simulink model "model_groundTethered"  (R2015b)
settings: Solver=ode45  StartTime=0.0  StopTime=T_sim  FixedStep=dt  RelTol=1e-3
PreLoadFcn:
  | setup;
InitFcn:
  | setup;
StartFcn:
  | setup;
values from neighbouring files (symbols this model uses):
  A_act = [-100 0 0 0 0 -100 0 0 0 0 -100 0 ... (16 elements, 4x4)]    [CD_spline.mat]    (also in CL_spline.mat; setup.m = -100*eye(4); setup_tmp_1p.m = -100*eye(4); setup_tmp_4p.m = -100*eye(4))
  A_init = [1.0386 0 12.9]    [CD_spline.mat]    (also in CL_spline.mat; setup_KiteModel_4points.m = Pc_init + d_n_r * w_k * w_rel * [-1;0;0])
  A_Kite = 7    [CD_spline.mat]    (also in CL_spline.mat; setup.m = 10.18; setup_tmp_1p.m = 10.18; setup_tmp_4p.m = 10.18)
  A_prd = [0 0 0 -640 0 0 0 0 0 0 -640 0 ... (36 elements, 6x6)]    [CD_spline.mat]    (also in CL_spline.mat; setup.m = 1000 * A_M_aug; setup_tmp_1p.m = 1000 * A_M_aug; setup_tmp_4p.m = 1000 * A_M_aug)
  A_ref = [0 0 0 -10000 0 0 0 0 0 0 -10000 0 ... (36 elements, 6x6)]    [CD_spline.mat]    (also in CL_spline.mat; setup.m = zeros(6); setup_tmp_1p.m = zeros(6); setup_tmp_4p.m = zeros(6))
  A_t_ref_cl = [0 0 0 -0.64 0 0 0 0 0 0 -0.64 0 ... (36 elements, 6x6)]    [CD_spline.mat]    (also in CL_spline.mat; setup.m = A_t_ref; setup_tmp_1p.m = A_t_ref; setup_tmp_4p.m = A_t_ref)
  alpha_0 = 10 * pi/180    (= 0.174532925199)    [setup_KiteModel_4points.m]
  alpha_s_0 = 10 * pi/180    (= 0.174532925199)    [setup_KiteModel_4points.m]
  ASideRel = 0    [CD_spline.mat]    (also in CL_spline.mat; setup.m; setup_tmp_1p.m; setup_tmp_4p.m = 0.306)
  B_act = [100 0 0 0 0 100 0 0 0 0 100 0 ... (16 elements, 4x4)]    [CD_spline.mat]    (also in CL_spline.mat; setup.m = 100*eye(4); setup_tmp_1p.m = 100*eye(4); setup_tmp_4p.m = 100*eye(4))
  B_init = [0 0 15.13]    [CD_spline.mat]    (also in CL_spline.mat; setup_KiteModel_4points.m = Pc_init + h_kite * [0;0;1;])
  B_ref = [0 0 0 10000 0 0 0 0 0 0 10000 0 ... (18 elements, 6x3)]    [CD_spline.mat]    (also in CL_spline.mat; setup.m = zeros(6,3); setup_tmp_1p.m = zeros(6,3); setup_tmp_4p.m = zeros(6,3))
  B_t_ref_cl = [0 0 0 0.64 0 0 0 0 0 0 0.64 0 ... (18 elements, 6x3)]    [CD_spline.mat]    (also in CL_spline.mat)
  Bpbl = [0 0 0 1 0 0 0 0 0 0 1 0 ... (18 elements, 6x3)]    [CD_spline.mat]    (also in CL_spline.mat; setup.m = [zeros(3); eye(3)]; setup_tmp_1p.m = [zeros(3); eye(3)]; setup_tmp_4p.m = [zeros(3); eye(3)])
  c0 = 614000    [CD_spline.mat]    (also in CL_spline.mat; setup.m; setup_tmp_1p.m; setup_tmp_4p.m)
  C_A = [0 0.3 -1e-06 1 -0.3 0 1e-06 1 0 -0.3 -1e-06 1 ... (16 elements, 4x4)]    [CD_spline.mat]    (also in CL_spline.mat; setup.m = [0, -R, 0, R; setup_tmp_1p.m = [0, -R, 0, R; setup_tmp_4p.m = [0, -R, 0, R)
  C_A_inv = [0 -1.66666666667 -1.23358113847e-17 1.66666666667 1.66666666667 2.46716227694e-17 -1.66666666667 0 -250000 250000 -250000 250000 ... (16 elements, 4x4)]    [CD_spline.mat]    (also in CL_spline.mat; setup.m = C_A \eye(4); setup_tmp_1p.m = C_A \eye(4); setup_tmp_4p.m = C_A \eye(4))
  C_D_Kite = 0.05    [CD_spline.mat]    (also in CL_spline.mat; setup.m = 0.005; setup_tmp_1p.m = 0.005)
  C_init = [0 2.5965 12.9]    [CD_spline.mat]    (also in CL_spline.mat; setup_KiteModel_4points.m = Pc_init + 0.5 * w_k * w_rel * [0;1;0])
  C_L_Kite = 0.1    [CD_spline.mat]    (also in CL_spline.mat; setup.m = 0.01; setup_tmp_1p.m = 0.01)
  CD_spline_coefs = CD_spline.coefs    [setup_KiteModel_4points.m]
  CD_tether = 0.96    [CD_spline.mat]    (also in CL_spline.mat; setup.m; setup_tmp_1p.m; setup_tmp_4p.m)
  CL_spline_coefs = CL_spline.coefs    [setup_KiteModel_4points.m]
  d0 = 473    [CD_spline.mat]    (also in CL_spline.mat; setup.m; setup_tmp_1p.m; setup_tmp_4p.m)
  D_init = [0 -2.5965 12.9]    [CD_spline.mat]    (also in CL_spline.mat; setup_KiteModel_4points.m = Pc_init - 0.5 * w_k * w_rel * [0;1;0])
  d_tether = 0.004    [CD_spline.mat]    (also in CL_spline.mat; setup.m; setup_tmp_1p.m; setup_tmp_4p.m)
  delta_dead = 0.5    [CD_spline.mat]    (also in CL_spline.mat; setup.m; setup_tmp_1p.m; setup_tmp_4p.m)
  e_0 = 0.01    [CD_spline.mat]    (also in CL_spline.mat; setup.m; setup_tmp_1p.m; setup_tmp_4p.m)
  epsilon = 0.6    [CD_spline.mat]    (also in CL_spline.mat; setup.m; setup_tmp_1p.m; setup_tmp_4p.m)
  eta_init = [0 0 0]    [CD_spline.mat]    (also in CL_spline.mat; setup.m = zeros(3,1); setup_tmp_1p.m = zeros(3,1); setup_tmp_4p.m = zeros(3,1))
  g = 9.81    [CD_spline.mat]    (also in CL_spline.mat; setup.m; setup_tmp_1p.m; setup_tmp_4p.m)
  g_vec = [0 0 9.81]    [CD_spline.mat]    (also in CL_spline.mat; setup.m = [0;0;9.81]; setup_tmp_1p.m = [0;0;9.81]; setup_tmp_4p.m = [0;0;9.81])
  Gamma_ad = 100    [CD_spline.mat]    (also in CL_spline.mat; setup.m = 100;100; setup_tmp_1p.m = 100;100; setup_tmp_4p.m = 100;100)
  Gamma_pred = 100    [CD_spline.mat]    (also in CL_spline.mat; setup.m; setup_tmp_1p.m; setup_tmp_4p.m)
  J = [0.018  0  0; 0  0.018  0; 0  0  0.009]    [CD_spline.mat]    (also in CL_spline.mat; setup.m = diag([Ixx, Iyy, Izz]); setup_tmp_1p.m = diag([Ixx, Iyy, Izz]); setup_tmp_4p.m = diag([Ixx, Iyy, Izz]))
  Jinv = [55.5555555556  0  0; 0  55.5555555556  0; 0  0  111.111111111]    [CD_spline.mat]    (also in CL_spline.mat; setup.m = J \ eye(3); setup_tmp_1p.m = J \ eye(3); setup_tmp_4p.m = J \ eye(3))
  K = 1 - ASideRel    [setup_KiteModel_4points.m]
  k_e_eta = 10000    [CD_spline.mat]    (also in CL_spline.mat; setup.m; setup_tmp_1p.m; setup_tmp_4p.m)
  k_e_eta_dot = 400    [CD_spline.mat]    (also in CL_spline.mat; setup.m; setup_tmp_1p.m; setup_tmp_4p.m)
  k_e_eta_I = 1    [CD_spline.mat]    (also in CL_spline.mat; setup.m; setup_tmp_1p.m; setup_tmp_4p.m)
  K_i_t = [10  0  0; 0  10  0; 0  0  10]    [CD_spline.mat]    (also in CL_spline.mat; setup.m = 10*eye(3); setup_tmp_1p.m = 10*eye(3); setup_tmp_4p.m = 10*eye(3))
  K_v_t = [1.6  0  0; 0  1.6  0; 0  0  1.6]    [CD_spline.mat]    (also in CL_spline.mat; setup.m = 2*omega_0_trans*zeta_0_trans*eye(3); setup_tmp_1p.m = 2*omega_0_trans*zeta_0_trans*eye(3); setup_tmp_4p.m = 2*omega_0_trans*zeta_0_trans*eye(3))
  K_x_t = [0.64  0  0; 0  0.64  0; 0  0  0.64]    [CD_spline.mat]    (also in CL_spline.mat; setup.m = omega_0_trans^2*eye(3); setup_tmp_1p.m = omega_0_trans^2*eye(3); setup_tmp_4p.m = omega_0_trans^2*eye(3))
  l_s0 = 1    [CD_spline.mat]    (also in CL_spline.mat; setup.m = 1.42857142857; setup_tmp_1p.m = 1.42857142857; setup_tmp_4p.m = 1.66666666667)
  l_s_BP = norm( B_init - p_B_UAV_init)    [setup_KiteModel_4points.m]
  l_s_PUav = norm( pos_UAV_init - p_B_UAV_init)    [setup_KiteModel_4points.m]
  ls_AB = norm( A_init -  B_init)    [setup_KiteModel_4points.m]
  ls_AC = norm( A_init -  C_init)    [setup_KiteModel_4points.m]
  ls_AD = norm( A_init -  D_init)    [setup_KiteModel_4points.m]
  ls_AKcu = norm( A_init -  P_kcu)    [setup_KiteModel_4points.m]
  ls_CB = norm( C_init -  B_init)    [setup_KiteModel_4points.m]
  ls_CD = norm( C_init -  D_init)    [setup_KiteModel_4points.m]
  ls_CKcu = norm( C_init - P_kcu)    [setup_KiteModel_4points.m]
  ls_DB = norm( D_init - B_init )    [setup_KiteModel_4points.m]
  ls_DKcu = norm( D_init - P_kcu)    [setup_KiteModel_4points.m]
  m_A = 3.29    [CD_spline.mat]    (also in CL_spline.mat; setup_KiteModel_4points.m = nose_mass_fraction * m_kite)
  m_B = 1.484    [CD_spline.mat]    (also in CL_spline.mat; setup_KiteModel_4points.m = 0.4 * (1-nose_mass_fraction)*m_kite)
  m_C = 1.113    [CD_spline.mat]    (also in CL_spline.mat; setup_KiteModel_4points.m = 0.3 * (1-nose_mass_fraction)*m_kite)
  m_D = 1.113    [CD_spline.mat]    (also in CL_spline.mat; setup_KiteModel_4points.m = 0.3 * (1-nose_mass_fraction)*m_kite)
  m_kite = 7    [CD_spline.mat]    (also in CL_spline.mat; setup.m = 5;7; setup_tmp_1p.m = 5;7; setup_tmp_4p.m = 6.21)
  m_p = 0.013    [CD_spline.mat]    (also in CL_spline.mat; setup.m = 0.0185714285714; setup_tmp_1p.m = 0.0185714285714; setup_tmp_4p.m = 0.0216666666667)
  m_uav = 3    [CD_spline.mat]    (also in CL_spline.mat; setup.m; setup_tmp_1p.m; setup_tmp_4p.m)
  n = 10    [CD_spline.mat]    (also in CL_spline.mat; setup.m; setup_tmp_1p.m; setup_tmp_4p.m)
  n_t_p = 7    [setup.m]    (also in setup_tmp_1p.m; setup_tmp_4p.m = 6)
  omega_init = [0 0 0]    [CD_spline.mat]    (also in CL_spline.mat; setup.m = zeros(3,1); setup_tmp_1p.m = zeros(3,1); setup_tmp_4p.m = zeros(3,1))
  p_B_UAV_init = B_init + [0;0;l_s0]    [setup_KiteModel_4points.m]
  p_init = [0 0 1 0 0 2 0 0 3 0 0 4 ... (30 elements, 30x1)]    [CD_spline.mat]    (also in CL_spline.mat; setup.m = zeros(3*n,1); setup_tmp_1p.m = zeros(3*n,1); setup_tmp_4p.m = zeros(3*n,1))
  p_init_4p = zeros(3*n_t_p,1)    [setup.m]    (also in setup_tmp_4p.m)
  P_prd = [712.5 0 0 156.25 0 0 0 712.5 0 0 156.25 0 ... (36 elements, 6x6)]    [CD_spline.mat]    (also in CL_spline.mat; setup.m = 1000 * P_tref; setup_tmp_1p.m = 1000 * P_tref; setup_tmp_4p.m = 1000 * P_tref)
  P_tref = [0.7125 0 0 0.15625 0 0 0 0.7125 0 0 0.15625 0 ... (36 elements, 6x6)]    [CD_spline.mat]    (also in CL_spline.mat; setup.m = lyap(A_M_aug', Q); setup_tmp_1p.m = lyap(A_M_aug', Q); setup_tmp_4p.m = lyap(A_M_aug', Q))
  pos_UAV_init = p_B_UAV_init + [0;0;l_s0]    [setup_KiteModel_4points.m]
  rho_air = 1.225    [CD_spline.mat]    (also in CL_spline.mat; setup.m; setup_tmp_1p.m; setup_tmp_4p.m)
  rho_t = 0.013    [CD_spline.mat]    (also in CL_spline.mat; setup.m; setup_tmp_1p.m; setup_tmp_4p.m)
  sample_log = 0.01    [CD_spline.mat]    (also in CL_spline.mat; setup.m; setup_tmp_1p.m; setup_tmp_4p.m)
  t0 = 1    [CD_spline.mat]    (also in CL_spline.mat; setup.m; setup_tmp_1p.m; setup_tmp_4p.m)
  t1 = 3    [CD_spline.mat]    (also in CL_spline.mat; setup.m; setup_tmp_1p.m; setup_tmp_4p.m)
  T_launch = 40    [CD_spline.mat]    (also in CL_spline.mat; setup.m; setup_tmp_1p.m; setup_tmp_4p.m)
  Theta_max = 60    [CD_spline.mat]    (also in CL_spline.mat; setup.m; setup_tmp_1p.m; setup_tmp_4p.m)
  Thrust_Max = 80    [CD_spline.mat]    (also in CL_spline.mat; setup.m = 1000000000; setup_tmp_1p.m = 100; setup_tmp_4p.m = 1000000000)
  Tx = 10    [CD_spline.mat]    (also in CL_spline.mat; setup.m; setup_tmp_1p.m; setup_tmp_4p.m)
  Ty = 10    [CD_spline.mat]    (also in CL_spline.mat; setup.m; setup_tmp_1p.m; setup_tmp_4p.m)
  Tz = 10    [CD_spline.mat]    (also in CL_spline.mat; setup.m; setup_tmp_1p.m; setup_tmp_4p.m = 15)
  v_w_vec = [1 1 1]    [CD_spline.mat]    (also in CL_spline.mat; setup.m = [0.1;0;0]; setup_tmp_1p.m = [1;0;0]; setup_tmp_4p.m = [3;0;0])
  x0num = 0    [CD_spline.mat]    (also in CL_spline.mat; polynomial_trajectory.m = double( solutions_x.x0 ))
  x1num = 0    [CD_spline.mat]    (also in CL_spline.mat; polynomial_trajectory.m = double( solutions_x.x1 ))
  x2num = 0    [CD_spline.mat]    (also in CL_spline.mat; polynomial_trajectory.m = double( solutions_x.x2 ))
  x3num = 0.05    [CD_spline.mat]    (also in CL_spline.mat; polynomial_trajectory.m = double( solutions_x.x3 ))
  x4num = -0.0075    [CD_spline.mat]    (also in CL_spline.mat; polynomial_trajectory.m = double( solutions_x.x4 ))
  x5num = 0.0003    [CD_spline.mat]    (also in CL_spline.mat; polynomial_trajectory.m = double( solutions_x.x5 ))
  x_drone_init = [0 0 10]    [CD_spline.mat]    (also in CL_spline.mat; setup.m = p_init(3*n-2:3*n); setup_KiteModel_4points.m = pos_UAV_init; setup_tmp_1p.m = p_init(3*n-2:3*n))
  xT = 5    [CD_spline.mat]    (also in CL_spline.mat; setup.m = 1; setup_tmp_1p.m = 10; setup_tmp_4p.m = 10)
  y0num = 0    [CD_spline.mat]    (also in CL_spline.mat; polynomial_trajectory.m = double( solutions_y.y0 ))
  y1num = 0    [CD_spline.mat]    (also in CL_spline.mat; polynomial_trajectory.m = double( solutions_y.y1 ))
  y2num = 0    [CD_spline.mat]    (also in CL_spline.mat; polynomial_trajectory.m = double( solutions_y.y2 ))
  y3num = 0.1    [CD_spline.mat]    (also in CL_spline.mat; polynomial_trajectory.m = double( solutions_y.y3 ))
  y4num = -0.015    [CD_spline.mat]    (also in CL_spline.mat; polynomial_trajectory.m = double( solutions_y.y4 ))
  y5num = 0.0006    [CD_spline.mat]    (also in CL_spline.mat; polynomial_trajectory.m = double( solutions_y.y5 ))
  yT = 10    [CD_spline.mat]    (also in CL_spline.mat; setup.m = 1; setup_tmp_1p.m = 0; setup_tmp_4p.m = 0)
  z0num = 10    [CD_spline.mat]    (also in CL_spline.mat; polynomial_trajectory.m = double( solutions_z.z0 ))
  z1num = 0    [CD_spline.mat]    (also in CL_spline.mat; polynomial_trajectory.m = double( solutions_z.z1 ))
  z2num = 0    [CD_spline.mat]    (also in CL_spline.mat; polynomial_trajectory.m = double( solutions_z.z2 ))
  z3num = 0.4    [CD_spline.mat]    (also in CL_spline.mat; polynomial_trajectory.m = double( solutions_z.z3 ))
  z4num = -0.06    [CD_spline.mat]    (also in CL_spline.mat; polynomial_trajectory.m = double( solutions_z.z4 ))
  z5num = 0.0024    [CD_spline.mat]    (also in CL_spline.mat; polynomial_trajectory.m = double( solutions_z.z5 ))
  zT = 50    [CD_spline.mat]    (also in CL_spline.mat; setup.m; setup_tmp_1p.m; setup_tmp_4p.m = 75)
libraries: simulink x1
(part 2 of 3)

== system model_groundTethered/Plant/Tether_Kite_Tether_UAV_Dynamics_1P/First_order_lag_Actuator ==
  Propeller_RPMs_CMD : Inport
  Actuator : Subsystem
  Selector : Selector  InputPortWidth=4  IndexOptions=Index vector (dialog)  Indices=[4]  OutputSizes=1
  Selector1 : Selector  InputPortWidth=4  IndexOptions=Index vector (dialog)  Indices=[1:3]  OutputSizes=1
  Moments : Outport
  Thrust : Outport  Port=2
  wires:
  Selector/1 -> Thrust/1
  Selector1/1 -> Moments/1
  Actuator/1(Thrust_Moments) -> Selector1/1, Selector/1
  Propeller_RPMs_CMD/1 -> Actuator/1(Propeller_RPMs_cmd)

== system model_groundTethered/Plant/Tether_Kite_Tether_UAV_Dynamics_1P/Kite_Model_1P ==
  note: UNDER CONSTRUCTION!
  x_p_dot : Inport
  launch_flag : Inport  Port=2
  x_p : Inport  Port=3
  v_w_vec : Inport  Port=4
  l_s : Inport  Port=5
  Kite_Model : MATLAB Function  TreatAsAtomicUnit=on
  x_kite : Selector  InputPortWidth=3*n  IndexOptions=Index vector (dialog)  Indices=[3*(n-2)-2:3*(n-2)]  OutputSizes=1
  xdot_Kite : Selector  InputPortWidth=3*n  IndexOptions=Index vector (dialog)  Indices=[3*(n-2)-2:3*(n-2)]  OutputSizes=1
  xdot_aboveKite : Selector  InputPortWidth=3*n  IndexOptions=Index vector (dialog)  Indices=[3*(n-1)-2:3*(n-1)]  OutputSizes=1
  xdot_belowKite : Selector  InputPortWidth=3*n  IndexOptions=Index vector (dialog)  Indices=[3*(n-3)-2:3*(n-3)]  OutputSizes=1
  xp_aboveKite : Selector  InputPortWidth=3*n  IndexOptions=Index vector (dialog)  Indices=[3*(n-1)-2:3*(n-1)]  OutputSizes=1
  xp_belowKite : Selector  InputPortWidth=3*n  IndexOptions=Index vector (dialog)  Indices=[3*(n-3)-2:3*(n-3)]  OutputSizes=1
  x_dotdot_kite : Outport
  wires:
  xdot_aboveKite/1 -> Kite_Model/6(xdot_aboveKite)
  xdot_belowKite/1 -> Kite_Model/8(xdot_belowKite)
  x_kite/1 -> Kite_Model/4(x_kite)
  xp_belowKite/1 -> Kite_Model/5(xp_belowKite)
  xp_aboveKite/1 -> Kite_Model/3(xp_aboveKite)
  x_p_dot/1 -> xdot_aboveKite/1, xdot_Kite/1, xdot_belowKite/1
  xdot_Kite/1 -> Kite_Model/7(xdot_kite)
  launch_flag/1 -> Kite_Model/1(launch_flag)
  v_w_vec/1 -> Kite_Model/2(v_w_vec)
  x_p/1 -> xp_aboveKite/1, x_kite/1, xp_belowKite/1
  Kite_Model/1(x_dotdot_kite) -> x_dotdot_kite/1
  l_s/1 -> Kite_Model/9(l_s)

== system model_groundTethered/Plant/Tether_Kite_Tether_UAV_Dynamics_1P/Tethermodel_Ground2Kite_1P ==
  x_dot : Inport
  x : Inport  Port=2
  v_w_vec : Inport  Port=3
  v_ro_set : Inport  Port=4
  l_s : Inport  Port=5
  Kite_p : Selector  InputPortWidth=3*n  IndexOptions=Index vector (dialog)  Indices=[3*(n-2)-2 : 3*(n-2)]  OutputSizes=1
  Kite_p1 : Selector  InputPortWidth=3*n  IndexOptions=Index vector (dialog)  Indices=[3*(n-2)-2 : 3*(n-2)]  OutputSizes=1
  Selector6 : Selector  InputPortWidth=3*n  IndexOptions=Index vector (dialog)  Indices=[1 : 3*(n-3)]  OutputSizes=1
  Tether_Ground2Kite : MATLAB Function  TreatAsAtomicUnit=on
  select_Tether_particles : Selector  InputPortWidth=3*n  IndexOptions=Index vector (dialog)  Indices=[1 : 3*(n-3)]  OutputSizes=1
  x_dotdot_TetherG2K : Outport
  l_tether : Outport  Port=2
  l_s_dot : Outport  Port=3
  wires:
  v_w_vec/1 -> Tether_Ground2Kite/3(v_w_vec)
  x_dot/1 -> Kite_p1/1, select_Tether_particles/1
  x/1 -> Kite_p/1, Selector6/1
  Tether_Ground2Kite/1(x_dotdot_TetherG2K) -> x_dotdot_TetherG2K/1
  Tether_Ground2Kite/2(l_tether) -> l_tether/1
  Tether_Ground2Kite/3(l_s_dot) -> l_s_dot/1
  l_s/1 -> Tether_Ground2Kite/5(l_s)
  v_ro_set/1 -> Tether_Ground2Kite/4(v_ro_set)
  select_Tether_particles/1 -> Tether_Ground2Kite/1(x_dot)
  Selector6/1 -> Tether_Ground2Kite/2(x)
  Kite_p1/1 -> Tether_Ground2Kite/7(xp_dot_kite)
  Kite_p/1 -> Tether_Ground2Kite/6(xp_kite)

== system model_groundTethered/Plant/Tether_Kite_Tether_UAV_Dynamics_1P/Tethermodel_Kite2UAV ==
  x_p_dot : Inport
  launch_flag : Inport  Port=2
  x_p : Inport  Port=3
  v_w_vec : Inport  Port=4
  Tether_Kite2UAV : MATLAB Function  TreatAsAtomicUnit=on
  drone : Selector  InputPortWidth=3*n  IndexOptions=Index vector (dialog)  Indices=[3*n-2:3*n]  OutputSizes=1
  drone1 : Selector  InputPortWidth=3*n  IndexOptions=Index vector (dialog)  Indices=[3*n-2:3*n]  OutputSizes=1
  kite : Selector  InputPortWidth=3*n  IndexOptions=Index vector (dialog)  Indices=[3*(n-2)-2:3*(n-2)]  OutputSizes=1
  kite1 : Selector  InputPortWidth=3*n  IndexOptions=Index vector (dialog)  Indices=[3*(n-2)-2:3*(n-2)]  OutputSizes=1
  particle : Selector  InputPortWidth=3*n  IndexOptions=Index vector (dialog)  Indices=[3*(n-1)-2:3*(n-1)]  OutputSizes=1
  particle1 : Selector  InputPortWidth=3*n  IndexOptions=Index vector (dialog)  Indices=[3*(n-1)-2:3*(n-1)]  OutputSizes=1
  x_dotdot_p : Outport
  wires:
  Tether_Kite2UAV/1(x_dotdot_p) -> x_dotdot_p/1
  launch_flag/1 -> Tether_Kite2UAV/1(launch_flag)
  drone/1 -> Tether_Kite2UAV/2(xp_above)
  x_p_dot/1 -> drone1/1, kite1/1, particle1/1
  kite1/1 -> Tether_Kite2UAV/7(xp_dot_below)
  particle1/1 -> Tether_Kite2UAV/6(xp_dot)
  particle/1 -> Tether_Kite2UAV/3(xp)
  drone1/1 -> Tether_Kite2UAV/5(xp_dot_above)
  x_p/1 -> kite/1, particle/1, drone/1
  kite/1 -> Tether_Kite2UAV/4(xp_below)
  v_w_vec/1 -> Tether_Kite2UAV/8(v_w_vec)

== system model_groundTethered/Plant/Tether_Kite_Tether_UAV_Dynamics_1P/UAV_Model ==
  x_p_dot : Inport
  x_p : Inport  Port=2
  u_M : Inport  Port=3
  u_Thrust_I : Inport  Port=4
  eta : Inport  Port=5
  omega : Inport  Port=6
  Kite1 : Selector  InputPortWidth=3*n  IndexOptions=Index vector (dialog)  Indices=[3*n-2:3*n]  OutputSizes=1
  Kite2 : Selector  InputPortWidth=3*n  IndexOptions=Index vector (dialog)  Indices=[3*n-2:3*n]  OutputSizes=1
  Rotate thrust vector according to attitude : MATLAB Function  TreatAsAtomicUnit=on
  To Workspace4 : ToWorkspace  VariableName=F_T_b  SaveFormat=Timeseries  SampleTime=sample_log
  UAV_Dynamics : MATLAB Function  TreatAsAtomicUnit=on
  particle1 : Selector  InputPortWidth=3*n  IndexOptions=Index vector (dialog)  Indices=[3*(n-1)-2:3*(n-1)]  OutputSizes=1
  particle2 : Selector  InputPortWidth=3*n  IndexOptions=Index vector (dialog)  Indices=[3*(n-1)-2:3*(n-1)]  OutputSizes=1
  x_dotdot_uav : Outport
  omega_dot : Outport  Port=2
  eta_dot : Outport  Port=3
  tag scope: disturbance=global
  wires:
  Rotate thrust vector according to attitude/1(u_Thrust_B) -> To Workspace4/1, UAV_Dynamics/1(Thrust)
  UAV_Dynamics/1(x_dotdot_uav_trans) -> x_dotdot_uav/1
  Kite1/1 -> UAV_Dynamics/2(x_UAV)
  x_p/1 -> Kite1/1, particle2/1
  particle1/1 -> UAV_Dynamics/5(x_dot_belowUAV)
  Kite2/1 -> UAV_Dynamics/4(x_dot_UAV)
  x_p_dot/1 -> particle1/1, Kite2/1
  particle2/1 -> UAV_Dynamics/3(x_below_UAV)
  UAV_Dynamics/4(disturbance) -> [disturbance]
  UAV_Dynamics/2(omega_dot) -> omega_dot/1
  UAV_Dynamics/3(eta_dot) -> eta_dot/1
  u_M/1 -> UAV_Dynamics/7(u_M)
  eta/1 -> Rotate thrust vector according to attitude/2(eta), UAV_Dynamics/8(eta)
  omega/1 -> UAV_Dynamics/6(omega)
  u_Thrust_I/1 -> Rotate thrust vector according to attitude/1(u_Thrust_I)

== system model_groundTethered/Plant/Tether_Kite_Tether_UAV_Dynamics_4P/First_order_lag_Actuator ==
  Propeller_RPMs_CMD : Inport
  Actuator : Subsystem
  Selector : Selector  InputPortWidth=4  IndexOptions=Index vector (dialog)  Indices=[4]  OutputSizes=1
  Selector1 : Selector  InputPortWidth=4  IndexOptions=Index vector (dialog)  Indices=[1:3]  OutputSizes=1
  Moments : Outport
  Thrust : Outport  Port=2
  wires:
  Selector/1 -> Thrust/1
  Selector1/1 -> Moments/1
  Actuator/1(Thrust_Moments) -> Selector1/1, Selector/1
  Propeller_RPMs_CMD/1 -> Actuator/1(Propeller_RPMs_cmd)

== system model_groundTethered/Plant/Tether_Kite_Tether_UAV_Dynamics_4P/Kite_Model_1P ==
  note: UNDER CONSTRUCTION!
  x_p_dot : Inport
  launch_flag : Inport  Port=2
  x_p : Inport  Port=3
  v_w_vec : Inport  Port=4
  l_s : Inport  Port=5
  Kite_Model : MATLAB Function  TreatAsAtomicUnit=on
  x_kite : Selector  InputPortWidth=3*n  IndexOptions=Index vector (dialog)  Indices=[3*(n-2)-2:3*(n-2)]  OutputSizes=1
  xdot_Kite : Selector  InputPortWidth=3*n  IndexOptions=Index vector (dialog)  Indices=[3*(n-2)-2:3*(n-2)]  OutputSizes=1
  xdot_aboveKite : Selector  InputPortWidth=3*n  IndexOptions=Index vector (dialog)  Indices=[3*(n-1)-2:3*(n-1)]  OutputSizes=1
  xdot_belowKite : Selector  InputPortWidth=3*n  IndexOptions=Index vector (dialog)  Indices=[3*(n-3)-2:3*(n-3)]  OutputSizes=1
  xp_aboveKite : Selector  InputPortWidth=3*n  IndexOptions=Index vector (dialog)  Indices=[3*(n-1)-2:3*(n-1)]  OutputSizes=1
  xp_belowKite : Selector  InputPortWidth=3*n  IndexOptions=Index vector (dialog)  Indices=[3*(n-3)-2:3*(n-3)]  OutputSizes=1
  x_dotdot_kite : Outport
  wires:
  xdot_aboveKite/1 -> Kite_Model/6(xdot_aboveKite)
  xdot_belowKite/1 -> Kite_Model/8(xdot_belowKite)
  x_kite/1 -> Kite_Model/4(x_kite)
  xp_belowKite/1 -> Kite_Model/5(xp_belowKite)
  xp_aboveKite/1 -> Kite_Model/3(xp_aboveKite)
  x_p_dot/1 -> xdot_aboveKite/1, xdot_Kite/1, xdot_belowKite/1
  xdot_Kite/1 -> Kite_Model/7(xdot_kite)
  launch_flag/1 -> Kite_Model/1(launch_flag)
  v_w_vec/1 -> Kite_Model/2(v_w_vec)
  x_p/1 -> xp_aboveKite/1, x_kite/1, xp_belowKite/1
  Kite_Model/1(x_dotdot_kite) -> x_dotdot_kite/1
  l_s/1 -> Kite_Model/9(l_s)

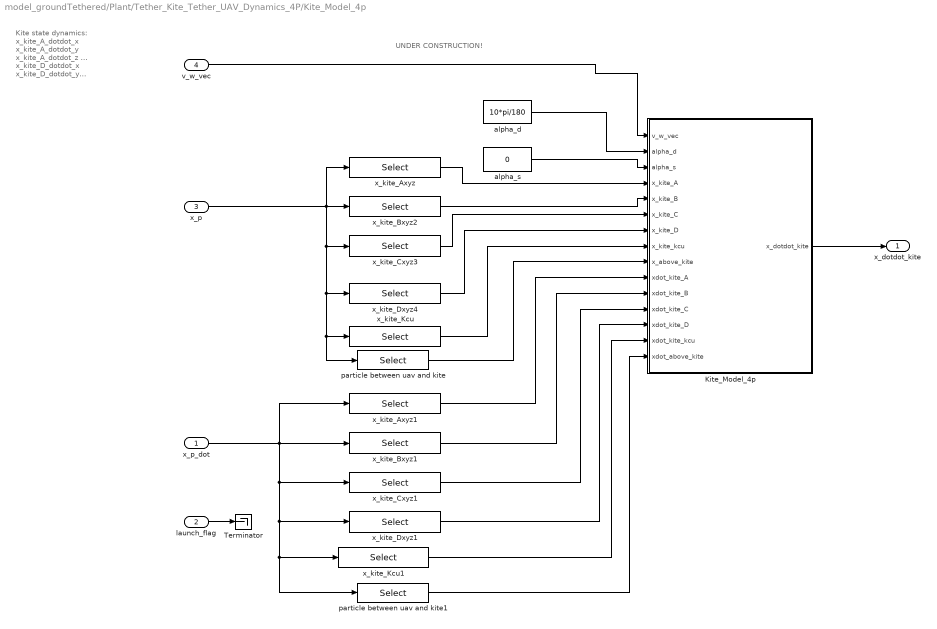
== system model_groundTethered/Plant/Tether_Kite_Tether_UAV_Dynamics_4P/Kite_Model_4p ==
  note: Kite state dynamics:
      |
      | x_kite_A_dotdot_x
      | x_kite_A_dotdot_y
      | x_kite_A_dotdot_z
      | ...
      | x_kite_D_dotdot_x
      | x_kite_D_dotdot_y
      | x_kite_D_dotdot_z
  note: UNDER CONSTRUCTION!
  x_p_dot : Inport
  launch_flag : Inport  Port=2
  x_p : Inport  Port=3
  v_w_vec : Inport  Port=4
  Kite_Model_4p : MATLAB Function  TreatAsAtomicUnit=on
  Terminator : Terminator
  alpha_d : Constant  Value=10*pi/180
  alpha_s : Constant  Value=0
  particle between uav and kite : Selector  InputPortWidth=3*n_t_p +18  IndexOptions=Index vector (dialog)  Indices=[3*n_t_p+13: 3*n_t_p+15]  OutputSizes=1
  particle between uav and kite1 : Selector  InputPortWidth=3*n_t_p +18  IndexOptions=Index vector (dialog)  Indices=[3*n_t_p+13: 3*n_t_p+15]  OutputSizes=1
  x_kite_Axyz : Selector  InputPortWidth=3*n_t_p + 18  IndexOptions=Index vector (dialog)  Indices=[3*n_t_p+1:3*n_t_p+3]  OutputSizes=1
  x_kite_Axyz1 : Selector  InputPortWidth=3*n_t_p + 18  IndexOptions=Index vector (dialog)  Indices=[3*n_t_p+1:3*n_t_p+3]  OutputSizes=1
  x_kite_Bxyz1 : Selector  InputPortWidth=3*n_t_p + 18  IndexOptions=Index vector (dialog)  Indices=[3*n_t_p+4:3*n_t_p+6]  OutputSizes=1
  x_kite_Bxyz2 : Selector  InputPortWidth=3*n_t_p + 18  IndexOptions=Index vector (dialog)  Indices=[3*n_t_p+4:3*n_t_p+6]  OutputSizes=1
  x_kite_Cxyz1 : Selector  InputPortWidth=3*n_t_p + 18  IndexOptions=Index vector (dialog)  Indices=[3*n_t_p+7:3*n_t_p+9]  OutputSizes=1
  x_kite_Cxyz3 : Selector  InputPortWidth=3*n_t_p + 18  IndexOptions=Index vector (dialog)  Indices=[3*n_t_p+7:3*n_t_p+9]  OutputSizes=1
  x_kite_Dxyz1 : Selector  InputPortWidth=3*n_t_p + 18  IndexOptions=Index vector (dialog)  Indices=[3*n_t_p+10:3*n_t_p+12]  OutputSizes=1
  x_kite_Dxyz4 : Selector  InputPortWidth=3*n_t_p + 18  IndexOptions=Index vector (dialog)  Indices=[3*n_t_p+10:3*n_t_p+12]  OutputSizes=1
  x_kite_Kcu : Selector  InputPortWidth=3*n_t_p +18  IndexOptions=Index vector (dialog)  Indices=[3*n_t_p-2:3*n_t_p]  OutputSizes=1
  x_kite_Kcu1 : Selector  InputPortWidth=3*n_t_p +18  IndexOptions=Index vector (dialog)  Indices=[3*n_t_p-2:3*n_t_p]  OutputSizes=1
  x_dotdot_kite : Outport
  wires:
  x_p_dot/1 -> particle between uav and kite1/1, x_kite_Kcu1/1, x_kite_Dxyz1/1, x_kite_Cxyz1/1, x_kite_Axyz1/1, x_kite_Bxyz1/1
  v_w_vec/1 -> Kite_Model_4p/1(v_w_vec)
  x_p/1 -> particle between uav and kite/1, x_kite_Kcu/1, x_kite_Dxyz4/1, x_kite_Cxyz3/1, x_kite_Bxyz2/1, x_kite_Axyz/1
  Kite_Model_4p/1(x_dotdot_kite) -> x_dotdot_kite/1
  alpha_d/1 -> Kite_Model_4p/2(alpha_d)
  alpha_s/1 -> Kite_Model_4p/3(alpha_s)
  x_kite_Axyz1/1 -> Kite_Model_4p/10(xdot_kite_A)
  x_kite_Bxyz1/1 -> Kite_Model_4p/11(xdot_kite_B)
  x_kite_Cxyz1/1 -> Kite_Model_4p/12(xdot_kite_C)
  x_kite_Dxyz1/1 -> Kite_Model_4p/13(xdot_kite_D)
  launch_flag/1 -> Terminator/1
  x_kite_Kcu1/1 -> Kite_Model_4p/14(xdot_kite_kcu)
  x_kite_Kcu/1 -> Kite_Model_4p/8(x_kite_kcu)
  x_kite_Dxyz4/1 -> Kite_Model_4p/7(x_kite_D)
  x_kite_Bxyz2/1 -> Kite_Model_4p/5(x_kite_B)
  x_kite_Axyz/1 -> Kite_Model_4p/4(x_kite_A)
  x_kite_Cxyz3/1 -> Kite_Model_4p/6(x_kite_C)
  particle between uav and kite/1 -> Kite_Model_4p/9(x_above_kite)
  particle between uav and kite1/1 -> Kite_Model_4p/15(xdot_above_kite)

== system model_groundTethered/Plant/Tether_Kite_Tether_UAV_Dynamics_4P/Tethermodel_Ground2Kite_4P ==
  x_dot : Inport
  x : Inport  Port=2
  v_w_vec : Inport  Port=3
  v_ro_set : Inport  Port=4
  l_s : Inport  Port=5
  Tether_Ground2Kite : MATLAB Function  TreatAsAtomicUnit=on
  select_Tether_particles : Selector  InputPortWidth=3*n_t_p+18  IndexOptions=Index vector (dialog)  Indices=[1 : 3*n_t_p]  OutputSizes=1
  select_Tether_particles1 : Selector  InputPortWidth=3*n_t_p+18  IndexOptions=Index vector (dialog)  Indices=[1 : 3*n_t_p]  OutputSizes=1
  x_kite_Axyz : Selector  InputPortWidth=3*n_t_p+18  IndexOptions=Index vector (dialog)  Indices=[3*n_t_p+1:3*n_t_p+3]  OutputSizes=1
  x_kite_Axyz1 : Selector  InputPortWidth=3*n_t_p+18  IndexOptions=Index vector (dialog)  Indices=[3*n_t_p+1:3*n_t_p+3]  OutputSizes=1
  x_kite_Cxyz1 : Selector  InputPortWidth=3*n_t_p+18  IndexOptions=Index vector (dialog)  Indices=[3*n_t_p+7:3*n_t_p+9]  OutputSizes=1
  x_kite_Cxyz3 : Selector  InputPortWidth=3*n_t_p+18  IndexOptions=Index vector (dialog)  Indices=[3*n_t_p+7:3*n_t_p+9]  OutputSizes=1
  x_kite_Dxyz1 : Selector  InputPortWidth=3*n_t_p+18  IndexOptions=Index vector (dialog)  Indices=[3*n_t_p+10:3*n_t_p+12]  OutputSizes=1
  x_kite_Dxyz4 : Selector  InputPortWidth=3*n_t_p+18  IndexOptions=Index vector (dialog)  Indices=[3*n_t_p+10:3*n_t_p+12]  OutputSizes=1
  x_dotdot_TetherG2K : Outport
  l_tether : Outport  Port=2
  l_s_dot : Outport  Port=3
  wires:
  v_w_vec/1 -> Tether_Ground2Kite/3(v_w_vec)
  x_dot/1 -> x_kite_Dxyz1/1, x_kite_Cxyz1/1, x_kite_Axyz1/1, select_Tether_particles/1
  x/1 -> x_kite_Dxyz4/1, x_kite_Cxyz3/1, x_kite_Axyz/1, select_Tether_particles1/1
  Tether_Ground2Kite/1(x_dotdot_TetherG2K) -> x_dotdot_TetherG2K/1
  Tether_Ground2Kite/2(l_tether) -> l_tether/1
  Tether_Ground2Kite/3(l_s_dot) -> l_s_dot/1
  l_s/1 -> Tether_Ground2Kite/5(l_s)
  v_ro_set/1 -> Tether_Ground2Kite/4(v_ro_set)
  select_Tether_particles/1 -> Tether_Ground2Kite/1(x_dot)
  select_Tether_particles1/1 -> Tether_Ground2Kite/2(x)
  x_kite_Axyz/1 -> Tether_Ground2Kite/6(x_kite_A)
  x_kite_Cxyz3/1 -> Tether_Ground2Kite/7(x_kite_C)
  x_kite_Dxyz4/1 -> Tether_Ground2Kite/8(x_kite_D)
  x_kite_Axyz1/1 -> Tether_Ground2Kite/9(xdot_kite_A)
  x_kite_Dxyz1/1 -> Tether_Ground2Kite/11(xdot_kite_D)
  x_kite_Cxyz1/1 -> Tether_Ground2Kite/10(xdot_kite_C)

== system model_groundTethered/Plant/Tether_Kite_Tether_UAV_Dynamics_4P/Tethermodel_Kite2UAV ==
  x_p_dot : Inport
  launch_flag : Inport  Port=2
  x_p : Inport  Port=3
  v_w_vec : Inport  Port=4
  Tether_Kite2UAV : MATLAB Function  TreatAsAtomicUnit=on
  f_T_above : Scope
  f_T_below : Scope
  particle between uav and kite : Selector  InputPortWidth=3*n_t_p +18  IndexOptions=Index vector (dialog)  Indices=[3*n_t_p+13: 3*n_t_p+15]  OutputSizes=1
  particle between uav and kite1 : Selector  InputPortWidth=3*n_t_p +18  IndexOptions=Index vector (dialog)  Indices=[3*n_t_p+13: 3*n_t_p+15]  OutputSizes=1
  uav : Selector  InputPortWidth=3*n_t_p +18  IndexOptions=Index vector (dialog)  Indices=[3*n_t_p + 16: 3*n_t_p + 18]  OutputSizes=1
  x_kite_B : Selector  InputPortWidth=3*n_t_p +18  IndexOptions=Index vector (dialog)  Indices=[3*n_t_p + 4: 3*n_t_p + 6]  OutputSizes=1
  x_kite_B1 : Selector  InputPortWidth=3*n_t_p +18  IndexOptions=Index vector (dialog)  Indices=[3*n_t_p + 4: 3*n_t_p + 6]  OutputSizes=1
  x_kite_B5 : Selector  InputPortWidth=3*n_t_p +18  IndexOptions=Index vector (dialog)  Indices=[3*n_t_p + 16: 3*n_t_p + 18]  OutputSizes=1
  x_dotdot_p : Outport
  wires:
  Tether_Kite2UAV/1(x_dotdot_p) -> x_dotdot_p/1
  launch_flag/1 -> Tether_Kite2UAV/1(launch_flag)
  uav/1 -> Tether_Kite2UAV/2(xp_above)
  x_kite_B1/1 -> Tether_Kite2UAV/7(xp_dot_below)
  x_p_dot/1 -> particle between uav and kite1/1, x_kite_B1/1, x_kite_B5/1
  particle between uav and kite/1 -> Tether_Kite2UAV/3(xp)
  x_kite_B5/1 -> Tether_Kite2UAV/5(xp_dot_above)
  x_p/1 -> uav/1, particle between uav and kite/1, x_kite_B/1
  x_kite_B/1 -> Tether_Kite2UAV/4(xp_below)
  v_w_vec/1 -> Tether_Kite2UAV/8(v_w_vec)
  particle between uav and kite1/1 -> Tether_Kite2UAV/6(xp_dot)
  Tether_Kite2UAV/2(f_T_below) -> f_T_below/1
  Tether_Kite2UAV/3(f_T_above) -> f_T_above/1

== system model_groundTethered/Plant/Tether_Kite_Tether_UAV_Dynamics_4P/UAV_Model ==
  x_p_dot : Inport
  x_p : Inport  Port=2
  u_M : Inport  Port=3
  u_Thrust_I : Inport  Port=4
  eta : Inport  Port=5
  omega : Inport  Port=6
  Kite1 : Selector  InputPortWidth=3*n_t_p + 18  IndexOptions=Index vector (dialog)  Indices=[3*n_t_p + 16:3*n_t_p + 18]  OutputSizes=1
  Kite2 : Selector  InputPortWidth=3*n_t_p + 18  IndexOptions=Index vector (dialog)  Indices=[3*n_t_p + 16:3*n_t_p + 18]  OutputSizes=1
  Kite3 : Selector  InputPortWidth=3*n_t_p + 18  IndexOptions=Index vector (dialog)  Indices=[3*n_t_p + 13:3*n_t_p + 15]  OutputSizes=1
  Kite4 : Selector  InputPortWidth=3*n_t_p + 18  IndexOptions=Index vector (dialog)  Indices=[3*n_t_p + 13:3*n_t_p + 15]  OutputSizes=1
  Rotate thrust vector according to attitude : MATLAB Function  TreatAsAtomicUnit=on
  To Workspace4 : ToWorkspace  VariableName=F_T_b  SaveFormat=Timeseries  SampleTime=sample_log
  UAV_Dynamics : MATLAB Function  TreatAsAtomicUnit=on
  x_dotdot_uav : Outport
  omega_dot : Outport  Port=2
  eta_dot : Outport  Port=3
  tag scope: disturbance=global
  wires:
  Rotate thrust vector according to attitude/1(u_Thrust_B) -> To Workspace4/1, UAV_Dynamics/1(Thrust)
  UAV_Dynamics/1(x_dotdot_uav_trans) -> x_dotdot_uav/1
  Kite1/1 -> UAV_Dynamics/2(x_UAV)
  Kite4/1 -> UAV_Dynamics/5(x_dot_belowUAV)
  Kite2/1 -> UAV_Dynamics/4(x_dot_UAV)
  x_p_dot/1 -> Kite4/1, Kite2/1
  x_p/1 -> Kite3/1, Kite1/1
  UAV_Dynamics/4(disturbance) -> [disturbance]
  UAV_Dynamics/2(omega_dot) -> omega_dot/1
  UAV_Dynamics/3(eta_dot) -> eta_dot/1
  u_M/1 -> UAV_Dynamics/7(u_M)
  eta/1 -> Rotate thrust vector according to attitude/2(eta), UAV_Dynamics/8(eta)
  omega/1 -> UAV_Dynamics/6(omega)
  u_Thrust_I/1 -> Rotate thrust vector according to attitude/1(u_Thrust_I)
  Kite3/1 -> UAV_Dynamics/3(x_below_UAV)

== system model_groundTethered/Controller/Outer_Loop_Position/Adaptive_Augmentation/Proj(Theta_hat, GammaY)_1column ==
  note: Ref.: Lavretsky, Robust and Adaptive Control, p. 329
      | Lecure Notes Nonlinear and Adaptive Control, TU Munich, FSD, SS2014, Robustness Modifications
  Theta_hat : Inport
  Theta_dot : Inport  Port=2
  Mux : Mux  Inputs=3
  Proj(Theta,Theta_dot) : MATLAB Function  TreatAsAtomicUnit=on
  Reshape1 : Reshape  OutputDimensionality=Row vector (2-D)
  Reshape2 : Reshape  OutputDimensionality=Row vector (2-D)
  To Workspace1 : ToWorkspace  VariableName=proj_flat  SaveFormat=Timeseries  SampleTime=sample_log
      settings: Save2DSignal=2-D array (concatenate along first dimension)
  To Workspace2 : ToWorkspace  VariableName=Theta_dot_save  SampleTime=sample_log
      settings: Save2DSignal=2-D array (concatenate along first dimension)
  To Workspace3 : ToWorkspace  VariableName=orthogonal_part  SampleTime=sample_log
      settings: Save2DSignal=2-D array (concatenate along first dimension)
  calculate_f : MATLAB Function  TreatAsAtomicUnit=on
  calculate_gradf : MATLAB Function  TreatAsAtomicUnit=on
  max_allowable_bound : Constant  Value=Theta_max
  projection_tolerance : Constant  Value=epsilon
  Theta_hat_dot : Outport
  wires:
  Proj(Theta,Theta_dot)/2(Theta_hat_dot_) -> Reshape1/1, Theta_hat_dot/1
  Proj(Theta,Theta_dot)/1(flag) -> Mux/2
  Proj(Theta,Theta_dot)/3(direction) -> Mux/3
  Mux/1 -> To Workspace1/1
  calculate_gradf/1(gradf) -> Proj(Theta,Theta_dot)/2(gradf)
  Theta_hat/1 -> calculate_gradf/1(theta_hat), calculate_f/1(theta_hat)
  projection_tolerance/1 -> calculate_f/3(epsilon), calculate_gradf/3(epsilon)
  max_allowable_bound/1 -> calculate_f/2(Theta_max), calculate_gradf/2(Theta_max)
  Theta_dot/1 -> Proj(Theta,Theta_dot)/3(Theta_dot)
  calculate_f/1(f) -> Mux/1, Proj(Theta,Theta_dot)/1(f)
  Reshape1/1 -> To Workspace2/1
  Proj(Theta,Theta_dot)/4(orthogonal_part) -> Reshape2/1
  Reshape2/1 -> To Workspace3/1

== system model_groundTethered/Controller/Outer_Loop_Position/Adaptive_Augmentation/Proj(Theta_hat, GammaY)_multicolumns ==
  note: Ref.: Lavretsky, Robust and Adaptive Control, p. 329
      | Lecure Notes Nonlinear and Adaptive Control, TU Munich, FSD, SS2014, Robustness Modifications
  Theta_hat : Inport
  Theta_dot : Inport  Port=2
  MATLAB Function : MATLAB Function  TreatAsAtomicUnit=on
  Matrix Concatenate : Concatenate  NumInputs=3  Mode=Multidimensional array
  Projection_Input_1 : Subsystem
  Projection_Input_2 : Subsystem
  Projection_Input_3 : Subsystem
  Theta_hat_dot : Outport
  wires:
  Theta_hat/1 -> MATLAB Function/1(Theta_hat)
  Theta_dot/1 -> MATLAB Function/2(Theta_hat_dot)
  Projection_Input_1/1(Out1) -> Matrix Concatenate/1
  MATLAB Function/1(Theta_hat_1) -> Projection_Input_1/1(In1)
  MATLAB Function/2(Theta_hat_dot_1) -> Projection_Input_1/2(In2)
  MATLAB Function/3(Theta_hat_2) -> Projection_Input_2/1(In1)
  MATLAB Function/4(Theta_hat_dot_2) -> Projection_Input_2/2(In2)
  MATLAB Function/6(Theta_hat_dot_3) -> Projection_Input_3/2(In2)
  MATLAB Function/5(Theta_hat_3) -> Projection_Input_3/1(In1)
  Projection_Input_2/1(Out1) -> Matrix Concatenate/2
  Projection_Input_3/1(Out1) -> Matrix Concatenate/3
  Matrix Concatenate/1 -> Theta_hat_dot/1

== system model_groundTethered/Controller/Outer_Loop_Position/Adaptive_Augmentation/Smooth_Deadzone_MRAC ==
  note: Ref.: Lavretsky, Robust and Adaptive Control, p. 319
  e : Inport
  Dead_Zone_Mod1 : Constant  Value=delta_dead
  Dead_Zone_Mod2 : Constant  Value=e_0
  Dot Product : DotProduct  InputSameDT=on  OutDataTypeStr=Inherit: Inherit via internal rule
  Mux : Mux  Inputs=2
  Sqrt : Sqrt  SaturateOnIntegerOverflow=on
  To Workspace8 : ToWorkspace  VariableName=e_ref_mu  SaveFormat=Timeseries  SampleTime=sample_log
      settings: Save2DSignal=2-D array (concatenate along first dimension)
  smooth_deadzone : MATLAB Function  TreatAsAtomicUnit=on
  mu_dead : Outport
  wires:
  e/1 -> Dot Product/1, Dot Product/2
  Dead_Zone_Mod1/1 -> smooth_deadzone/2(delta_dead)
  Dead_Zone_Mod2/1 -> smooth_deadzone/3(e_0)
  Dot Product/1 -> Sqrt/1
  Sqrt/1 -> Mux/1, smooth_deadzone/1(e_norm)
  smooth_deadzone/1(mu_dead) -> Mux/2, mu_dead/1
  Mux/1 -> To Workspace8/1

== system model_groundTethered/Controller/Outer_Loop_Position/Adaptive_Augmentation/Smooth_Deadzone_PMRAC ==
  note: Ref.: Lavretsky, Robust and Adaptive Control, p. 319
  e : Inport
  Dead_Zone_Mod1 : Constant  Value=delta_dead
  Dead_Zone_Mod2 : Constant  Value=e_0
  Dot Product : DotProduct  InputSameDT=on  OutDataTypeStr=Inherit: Inherit via internal rule
  Mux1 : Mux  Inputs=2
  Sqrt : Sqrt  SaturateOnIntegerOverflow=on
  To Workspace1 : ToWorkspace  VariableName=e_pref_mu  SaveFormat=Timeseries  SampleTime=sample_log
      settings: Save2DSignal=2-D array (concatenate along first dimension)
  smooth_deadzone : MATLAB Function  TreatAsAtomicUnit=on
  mu_dead : Outport
  wires:
  Dot Product/1 -> Sqrt/1
  Dead_Zone_Mod2/1 -> smooth_deadzone/3(e_0)
  Dead_Zone_Mod1/1 -> smooth_deadzone/2(delta_dead)
  e/1 -> Dot Product/2, Dot Product/1
  Sqrt/1 -> Mux1/1, smooth_deadzone/1(e_norm)
  smooth_deadzone/1(mu_dead) -> Mux1/2, mu_dead/1
  Mux1/1 -> To Workspace1/1

== system model_groundTethered/Plant/Tether_Kite_Tether_UAV_Dynamics_1P/First_order_lag_Actuator/Actuator ==
  Propeller_RPMs_cmd : Inport
  Add : Sum  Inputs=+-
  Gain : Gain  Gain=B_act  Multiplication=Matrix(K*u)
  Gain1 : Gain  Gain=A_act  Multiplication=Matrix(K*u)
  Integrator Limited1 : Integrator  InitialCondition=zeros(4,1)  LimitOutput=on  UpperSaturationLimit=Thrust_Max  LowerSaturationLimit=-Thrust_Max
  Output_Actuator : Gain  Gain=C_A  Multiplication=Matrix(K*u)
  Reaction_Deficit_Actuators : Scope
  Sum : Sum  Inputs=|++
  To Workspace1 : ToWorkspace  VariableName=prop_thrust_cmd  SaveFormat=Timeseries  SampleTime=sample_log
  To Workspace2 : ToWorkspace  VariableName=prop_thrust_real  SaveFormat=Timeseries  SampleTime=sample_log
  Thrust_Moments : Outport
  wires:
  Output_Actuator/1 -> Thrust_Moments/1
  Gain/1 -> Sum/1
  Gain1/1 -> Sum/2
  Sum/1 -> Integrator Limited1/1
  Propeller_RPMs_cmd/1 -> Add/1, To Workspace1/1, Gain/1
  Add/1 -> Reaction_Deficit_Actuators/1
  Integrator Limited1/1 -> Add/2, To Workspace2/1, Gain1/1, Output_Actuator/1

== system model_groundTethered/Plant/Tether_Kite_Tether_UAV_Dynamics_4P/First_order_lag_Actuator/Actuator ==
  Propeller_RPMs_cmd : Inport
  Add : Sum  Inputs=+-
  Gain : Gain  Gain=B_act  Multiplication=Matrix(K*u)
  Gain1 : Gain  Gain=A_act  Multiplication=Matrix(K*u)
  Integrator Limited1 : Integrator  InitialCondition=zeros(4,1)  LimitOutput=on  UpperSaturationLimit=Thrust_Max  LowerSaturationLimit=-Thrust_Max
  Output_Actuator : Gain  Gain=C_A  Multiplication=Matrix(K*u)
  Reaction_Deficit_Actuators : Scope
  Sum : Sum  Inputs=|++
  To Workspace1 : ToWorkspace  VariableName=prop_thrust_cmd  SaveFormat=Timeseries  SampleTime=sample_log
  To Workspace2 : ToWorkspace  VariableName=prop_thrust_real  SaveFormat=Timeseries  SampleTime=sample_log
  Thrust_Moments : Outport
  wires:
  Output_Actuator/1 -> Thrust_Moments/1
  Gain/1 -> Sum/1
  Gain1/1 -> Sum/2
  Sum/1 -> Integrator Limited1/1
  Propeller_RPMs_cmd/1 -> Add/1, To Workspace1/1, Gain/1
  Add/1 -> Reaction_Deficit_Actuators/1
  Integrator Limited1/1 -> Add/2, To Workspace2/1, Gain1/1, Output_Actuator/1

== system model_groundTethered/Controller/Outer_Loop_Position/Adaptive_Augmentation/Proj(Theta_hat, GammaY)_multicolumns/Projection_Input_1 ==
  In1 : Inport
  In2 : Inport  Port=2
  Proj(Theta,Theta_dot) : MATLAB Function  TreatAsAtomicUnit=on
  calculate_f : MATLAB Function  TreatAsAtomicUnit=on
  calculate_gradf : MATLAB Function  TreatAsAtomicUnit=on
  max_allowable_bound : Constant  Value=Theta_max
  projection_tolerance : Constant  Value=epsilon
  Out1 : Outport
  wires:
  calculate_f/1(f) -> Proj(Theta,Theta_dot)/1(f)
  In2/1 -> Proj(Theta,Theta_dot)/3(Theta_dot)
  max_allowable_bound/1 -> calculate_f/2(Theta_max), calculate_gradf/2(Theta_max)
  projection_tolerance/1 -> calculate_f/3(epsilon), calculate_gradf/3(epsilon)
  In1/1 -> calculate_gradf/1(theta_hat), calculate_f/1(theta_hat)
  calculate_gradf/1(gradf) -> Proj(Theta,Theta_dot)/2(gradf)
  Proj(Theta,Theta_dot)/1(Theta_hat_dot_) -> Out1/1

== system model_groundTethered/Controller/Outer_Loop_Position/Adaptive_Augmentation/Proj(Theta_hat, GammaY)_multicolumns/Projection_Input_2 ==
  In1 : Inport
  In2 : Inport  Port=2
  Proj(Theta,Theta_dot) : MATLAB Function  TreatAsAtomicUnit=on
  calculate_f : MATLAB Function  TreatAsAtomicUnit=on
  calculate_gradf : MATLAB Function  TreatAsAtomicUnit=on
  max_allowable_bound : Constant  Value=Theta_max
  projection_tolerance : Constant  Value=epsilon
  Out1 : Outport
  wires:
  calculate_f/1(f) -> Proj(Theta,Theta_dot)/1(f)
  In2/1 -> Proj(Theta,Theta_dot)/3(Theta_dot)
  max_allowable_bound/1 -> calculate_f/2(Theta_max), calculate_gradf/2(Theta_max)
  projection_tolerance/1 -> calculate_f/3(epsilon), calculate_gradf/3(epsilon)
  In1/1 -> calculate_gradf/1(theta_hat), calculate_f/1(theta_hat)
  calculate_gradf/1(gradf) -> Proj(Theta,Theta_dot)/2(gradf)
  Proj(Theta,Theta_dot)/1(Theta_hat_dot_) -> Out1/1

== system model_groundTethered/Controller/Outer_Loop_Position/Adaptive_Augmentation/Proj(Theta_hat, GammaY)_multicolumns/Projection_Input_3 ==
  In1 : Inport
  In2 : Inport  Port=2
  Mux : Mux  Inputs=3
  Proj(Theta,Theta_dot) : MATLAB Function  TreatAsAtomicUnit=on
  Scope : Scope
  Scope1 : Scope
  To Workspace1 : ToWorkspace  VariableName=proj_flat  SaveFormat=Timeseries  SampleTime=sample_log
      settings: Save2DSignal=2-D array (concatenate along first dimension)
  calculate_f : MATLAB Function  TreatAsAtomicUnit=on
  calculate_gradf : MATLAB Function  TreatAsAtomicUnit=on
  max_allowable_bound : Constant  Value=Theta_max
  projection_tolerance : Constant  Value=epsilon
  Out1 : Outport
  wires:
  calculate_f/1(f) -> Mux/1, Proj(Theta,Theta_dot)/1(f)
  In2/1 -> Proj(Theta,Theta_dot)/3(Theta_dot)
  max_allowable_bound/1 -> calculate_f/2(Theta_max), calculate_gradf/2(Theta_max)
  projection_tolerance/1 -> calculate_f/3(epsilon), calculate_gradf/3(epsilon)
  In1/1 -> calculate_gradf/1(theta_hat), calculate_f/1(theta_hat)
  calculate_gradf/1(gradf) -> Proj(Theta,Theta_dot)/2(gradf)
  Proj(Theta,Theta_dot)/2(Theta_hat_dot_) -> Out1/1
  Mux/1 -> To Workspace1/1
  Proj(Theta,Theta_dot)/3(direction) -> Scope/1, Mux/3
  Proj(Theta,Theta_dot)/1(flag) -> Scope1/1, Mux/2

== matlab function model_groundTethered/Controller/Inner_Loop_Attitude/Plant_Inversion_RD2/Plant_Inversion ==
  data: omega input; u_NDI output; eta input; eta_dot input; J input; nu_tot input
function u_NDI = fcn(omega, eta, eta_dot, J, nu_tot)
%#codegen
p = omega(1); 
q = omega(2); 
r = omega(3); 
Ix = J(1,1); 
Iy = J(2,2); 
Iz = J(3,3); 


cross_coupling = [ Iy*q*r - Iz*q*r
 Iz*p*r - Ix*p*r;
 Ix*p*q - Iy*p*q];

% T_inv = [1, sin(eta(1)) * tan(eta(2)), cos(eta(1)) * tan(eta(2)) ; 
% 0, cos(eta(1)), -sin(eta(1)); 
% 0, sin(eta(1))/cos(eta(2)), cos(eta(1))/cos(eta(2))] \ eye(3); 

T_inv = [1, 0, -sin(eta(2));
         0, cos(eta(1)), sin(eta(1))*cos(eta(2));
         0, -sin(eta(1)), cos(eta(1))*cos(eta(2))];
     
T_dot = eta_dot(1) * [0, cos(eta(1)) * tan(eta(2)), -sin(eta(1))*tan(eta(2)); 
                      0, -sin(eta(1)), -cos(eta(1));
                      0, cos(eta(1))/cos(eta(2)), -sin(eta(1))/cos(eta(2))]+...
        eta_dot(2) * [0, sin(eta(1))/cos(eta(2))^2, cos(eta(1))/cos(eta(2))^2; 
                       0, 0, 0; 
                       0, sin(eta(1))*sin(eta(2))/cos(eta(2))^2, cos(eta(1))*sin(eta(2))/cos(eta(2))^2];
                          
u_NDI = -cross_coupling + J * T_inv * ( -T_dot * omega + nu_tot);

== matlab function model_groundTethered/Flight_Path_Planner/Reference_Dynamic_x1 ==
  data: t input; y_ref output; y0num parameter; y1num parameter; y2num parameter; y3num parameter; y4num parameter; y5num parameter; yT parameter; Ty parameter
function y_ref = fcn(t,y0num, y1num, y2num, y3num, y4num, y5num, yT,Ty )

if t >= Ty
    y_ref = yT;
else
    y_ref = y5num * t^5 + y4num * t^4 + y3num * t^3 + y2num * t^2 + y1num * t + y0num;
end

== matlab function model_groundTethered/Flight_Path_Planner/Reference_Dynamic_x3 ==
  data: t input; x_ref output; x0num parameter; x1num parameter; x2num parameter; x3num parameter; x4num parameter; x5num parameter; Tx parameter; xT parameter
function x_ref = fcn(t,x0num, x1num, x2num, x3num, x4num, x5num, Tx,xT )

if t >= Tx
    x_ref = xT;
else
    x_ref = x5num * t^5 + x4num * t^4 + x3num * t^3 + x2num * t^2 + x1num * t + x0num;
end

== matlab function model_groundTethered/Flight_Path_Planner2/Reference_Dynamic_x ==
  data: x_cmd input; x_ref input; x_ref_dot output; t0 parameter; t1 parameter
function x_ref_dot = fcn(x_cmd, x_ref, t0, t1)

% a0 = 1;
% a1 = 5;

x_ref_dot = [0,1;
                -t0, -t1]*x_ref + [0;t0] * x_cmd;

== matlab function model_groundTethered/Controller/Inner_Loop_Attitude/estimate_eta_dot ==
  data: omega input; eta input; eta_dot output
function eta_dot  = fcn( omega, eta)
%#codegen

eta_dot = [1, sin(eta(1)) * tan(eta(2)), cos(eta(1)) * tan(eta(2)) ; 
0, cos(eta(1)), -sin(eta(1)); 
0, sin(eta(1))/cos(eta(2)), cos(eta(1))/cos(eta(2))] * omega;

== matlab function model_groundTethered/Flight_Path_Planner/Reference_Dynamic_x2 ==
  data: t input; z_ref output; z0num parameter; z1num parameter; z2num parameter; z3num parameter; z4num parameter; z5num parameter; Tz parameter; zT parameter
function z_ref = fcn(t,z0num, z1num, z2num, z3num, z4num, z5num,Tz, zT)

if t >= Tz
    z_ref = zT;
else
    z_ref = z5num * t^5 + z4num * t^4 + z3num * t^3 + z2num * t^2 + z1num * t + z0num;
end

== matlab function model_groundTethered/Controller/Outer_Loop_Position/Adaptive_Augmentation/Smooth_Deadzone_PMRAC/smooth_deadzone ==
  data: e_norm input; mu_dead output; delta_dead input; e_0 input
function mu_dead = fcn(e_norm, delta_dead, e_0)
%#codegen

mu_dead = max( 0, min( 1, (e_norm - delta_dead*e_0)/...
                          ( (1-delta_dead) * e_0) ) );

== matlab function model_groundTethered/Plant/Tether_Kite_Tether_UAV_Dynamics_4P/Kite_Model_1P/Kite_Model ==
  data: launch_flag input; x_dotdot_kite output; rho_air parameter; A_Kite parameter; g_vec parameter; C_L_Kite parameter; C_D_Kite parameter; m_kite parameter; v_w_vec input; ASideRel parameter; xp_aboveKite input; x_kite input; xp_belowKite input; xdot_aboveKite input; xdot_kite input; xdot_belowKite input; l_s input; c0 parameter; d0 parameter; l_s0 parameter
function x_dotdot_kite  = fcn(launch_flag,...
    rho_air, A_Kite, g_vec, C_L_Kite, C_D_Kite, m_kite, v_w_vec, ASideRel,...
    xp_aboveKite, x_kite, xp_belowKite,xdot_aboveKite, xdot_kite,...
    xdot_belowKite, l_s, c0, d0, l_s0)

c = c0/l_s;
d = d0/l_s;

% Tether forces from below and above
f_T_below = calcSpringDamperForce(c, norm(x_kite-xp_belowKite) , l_s, d, x_kite - xp_belowKite, xdot_kite - xdot_belowKite, 1 );
f_T_above = calcSpringDamperForce(c0, norm(xp_aboveKite-x_kite), l_s0, d0, xp_aboveKite-x_kite, xdot_aboveKite - xdot_kite, 1 );

% Calculate the apparent wind speed
v_a_k = v_w_vec - xdot_kite;
if launch_flag
    C_L_Kite = 0.5;
    C_D_Kite = 0.2;
end

[L_kite, D_kite, S_kite] = calcKiteForces(x_kite, xp_belowKite, ...
                                        v_a_k, C_L_Kite, rho_air, A_Kite, C_D_Kite, ASideRel);
m_kite = 0.1;
if launch_flag % kite is launched
    x_dotdot_kite = 1/m_kite * ( -f_T_below  - m_kite*g_vec  ... % remove the conection to 'drone tether'
        + D_kite + L_kite + 0*S_kite ) ;  % Kite dynamics
else
    x_dotdot_kite = 1/m_kite * ( -f_T_below + f_T_above - m_kite*g_vec  ...
        + 0*D_kite + 0*L_kite  + 0*S_kite);  % Kite dynamics
end

== matlab function model_groundTethered/Controller/Outer_Loop_Position/Predictor_Model_Translational_Dynamics/Reference_Model_Position ==
  data: A_prd input; A_ref input; x_prd_dotdot output; B_ref input; x_cmd input; x_p input; x_prd input
function x_prd_dotdot  = fcn(A_prd,A_ref,B_ref, x_cmd,x_p,x_prd)

    x_prd_dotdot = A_prd * (x_prd - x_p) + A_ref * x_p + B_ref * x_cmd;

== matlab function model_groundTethered/Controller/Outer_Loop_Position/Reference_Model_Translational_Dynamics/Reference_Model_Position ==
  data: A_t_ref_cl input; x_ref_dotdot output; B_t_ref input; x_cmd input; x_ref input
function x_ref_dotdot  = fcn(A_t_ref_cl,B_t_ref, x_cmd,x_ref)

    x_ref_dotdot = A_t_ref_cl * x_ref + B_t_ref * x_cmd;

== matlab function model_groundTethered/Controller/Outer_Loop_Position/Adaptive_Augmentation/Proj(Theta_hat, GammaY)_multicolumns/MATLAB Function ==
  data: Theta_hat input; Theta_hat_1 output; Theta_hat_dot_1 output; Theta_hat_dot input; Theta_hat_2 output; Theta_hat_dot_2 output; Theta_hat_3 output; Theta_hat_dot_3 output
function [Theta_hat_1,Theta_hat_dot_1, Theta_hat_2, Theta_hat_dot_2,...
            Theta_hat_3, Theta_hat_dot_3] = fcn(Theta_hat, Theta_hat_dot)
%#codegen
Theta_hat_1 = Theta_hat(1,:);
Theta_hat_2 = Theta_hat(2,:);
Theta_hat_3 = Theta_hat(3,:);

Theta_hat_dot_1 = Theta_hat_dot(1,:); 
Theta_hat_dot_2 = Theta_hat_dot(2,:);
Theta_hat_dot_3 = Theta_hat_dot(3,:);

== matlab function model_groundTethered/Controller/Outer_Loop_Position/Adaptive_Augmentation/Proj(Theta_hat, GammaY)_multicolumns/Projection_Input_1/Proj(Theta,Theta_dot) ==
  data: f input; gradf input; Theta_dot input; Theta_hat_dot_ output
function  Theta_hat_dot_ = fcn(f, gradf, Theta_dot )
%#codegen


if ( f > 0 && gradf*Theta_dot' > 0 )
    Theta_hat_dot_ = Theta_dot - f * ( (gradf'*gradf) / (gradf*gradf') * Theta_dot' )'   ;
else
    Theta_hat_dot_ =  Theta_dot;
end

== matlab function model_groundTethered/Controller/Outer_Loop_Position/Total_Thrust ==
  data: T_ref input; T_tot output
function T_tot  = fcn(T_ref)

%T_z = [0;0;norm(T_ref)];
T_tot = norm(T_ref);

== matlab function model_groundTethered/Controller/Outer_Loop_Position/Adaptive_Augmentation/Proj(Theta_hat, GammaY)_multicolumns/Projection_Input_1/calculate_f ==
  data: theta_hat input; f output; Theta_max input; epsilon input
function f   = fcn(theta_hat,Theta_max, epsilon )
%#codegen
f = ( (1+epsilon)*norm(theta_hat)^2 - (Theta_max)^2 ) / (epsilon*(Theta_max)^2);
